simulink model "steamjacket"  (R2018b)
settings: Solver=VariableStepAuto  StartTime=0.0  StopTime=10.0  RelTol=1e-3
settings Model: Creator=sofi  LastModifiedBy=art58

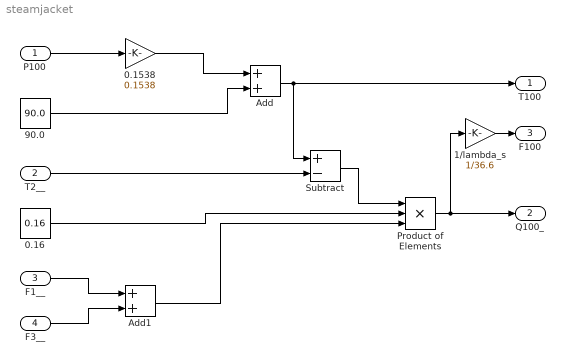
== system steamjacket ==
  P100 : Inport
  T2__ : Inport  Port=2
  F1__ : Inport  Port=3
  F3__ : Inport  Port=4
  0.1538 : Gain  Gain=0.1538
  0.16 : Constant  Value=0.16
  1/lambda_s : Gain  Gain=1/36.6
  90.0 : Constant  Value=90.0
  Add : Sum
  Add1 : Sum
  Product of Elements : Product  Inputs=***
  Subtract : Sum  Inputs=+-
  T100 : Outport
  Q100_ : Outport  Port=2
  F100 : Outport  Port=3
  wires:
  0.1538/1 -> Add/1
  P100/1 -> 0.1538/1
  90.0/1 -> Add/2
  Add/1 -> Subtract/1, T100/1
  Product of Elements/1 -> 1/lambda_s/1, Q100_/1
  Subtract/1 -> Product of Elements/1
  T2__/1 -> Subtract/2
  0.16/1 -> Product of Elements/2
  F1__/1 -> Add1/1
  F3__/1 -> Add1/2
  Add1/1 -> Product of Elements/3
  1/lambda_s/1 -> F100/1
